simulink model "lfo"  (R2018a)
settings: Solver=FixedStepDiscrete  StartTime=0.0  StopTime=30.0  RelTol=1e-3
libraries: dspsrcs4 x1
settings Model: Creator=Lu  LastModifiedBy=Lu
settings DataIOCC: SaveOutput=off  SaveTime=off
settings OptimizationCC: BlockReduction=off  ConditionallyExecuteInputs=off  DefaultParameterBehavior=Inlined
settings DebuggingCC: AlgebraicLoopMsg=error  SingleTaskRateTransMsg=error
settings HardwareCC: ProdBitPerPointer=32  ProdBitPerSizeT=32  ProdBitPerPtrDiffT=32  ProdLargestAtomicFloat=None  ProdIntDivRoundTo=Undefined  ProdEndianess=Unspecified  ProdWordSize=32  ProdHWDeviceType=ASIC/FPGA->ASIC/FPGA  TargetBitPerPointer=64  TargetBitPerSizeT=64  TargetBitPerPtrDiffT=64  TargetLongLongMode=on  TargetIntDivRoundTo=Zero  TargetEndianess=LittleEndian  TargetWordSize=64  TargetHWDeviceType=Custom Processor->MATLAB Host Computer  ProdEqTarget=off

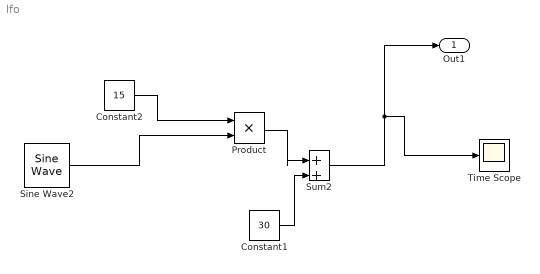
== system lfo ==
  Constant1 : Constant  Value=30  OutDataTypeStr=fixdt(1,16)
  Constant2 : Constant  Value=15  OutDataTypeStr=fixdt(1,8)
  Product : Product  OutMin=[-15]  OutMax=[15]  OutDataTypeStr=fixdt(1,16)  SaturateOnIntegerOverflow=on
  Sine Wave2 : dspsrcs4/Sine Wave  Amplitude=1  Frequency=0.5  Phase=0  SampleMode=Discrete  OutComplex=Real  CompMethod=Table lookup  TableSize=Memory  SampleTime=1/44100  SamplesPerFrame=1  ResetState=Restart at time zero  OutputFrames=off  dataType=Fixed-point  wordLen=8  udDataType=sfix(16)  fracBitsMode=Best precision  numFracBits=6  OutDataTypeStr=fixdt(1,8)  LastOutDataTypeStr=fixdt(1,8)
  Sum2 : Sum  Inputs=|++  AccumDataTypeStr=fixdt(1,16,0)  RndMeth=Ceiling  SaturateOnIntegerOverflow=on
  Time Scope : Scope
  Out1 : Outport  OutDataTypeStr=int16  PortDimensions=[1 1]  SampleTime=[2.2675736961451248e-05,0]
  wires:
  Constant1/1 -> Sum2/2
  Product/1 -> Sum2/1
  Sine Wave2/1 -> Product/2
  Constant2/1 -> Product/1
  Sum2/1 -> Out1/1, Time Scope/1
